simulink model "vehicle_svpwm"  (R2021a)
settings: Solver=VariableStepAuto  StartTime=0  StopTime=50  RelTol=1e-3
values from neighbouring files (symbols this model uses):
  Ld = 0.3e-3    (= 0.0003)    [PMSM_paramaters.m]
  Lq = 0.4e-3    (= 0.0004)    [PMSM_paramaters.m]
  P = 4    [PMSM_paramaters.m]
  Pm = 0.15    [PMSM_paramaters.m]
  Rs = 0.03    [PMSM_paramaters.m]
  T_lookup = [289,289,0]    [PMSM_paramaters.m]
  Torque = 289    [PMSM_paramaters.m]
  Ts = 1e-2    (= 0.01)    [PMSM_paramaters.m]
undefined symbols (not defined in the file or in its folder): sigbuilder_block
libraries: spsSeriesRLCBranchLib x18, spsMosfetLib x8, simulink x7, spsCurrentMeasurementLib x6, spsVoltageMeasurementLib x4, spsDCVoltageSourceLib x3, spsGroundLib x3, pid_lib x3, spsDiodeLib x2, spsRMSLib x2, autolibshared x1, spsTriangleGeneratorLib x1
(part 2 of 2)

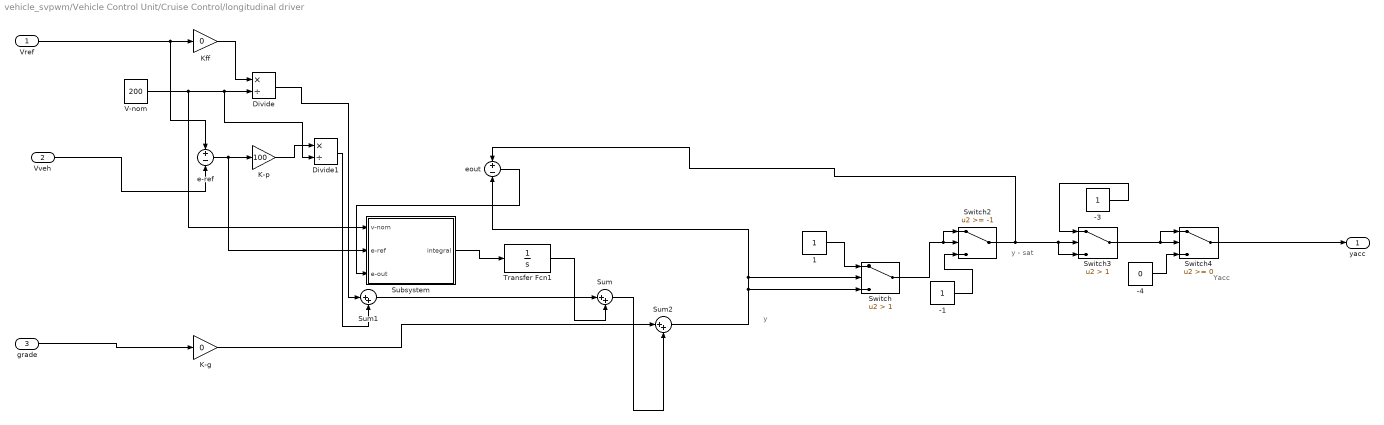
== system vehicle_svpwm/Vehicle Control Unit/Cruise Control/longitudinal driver ==
  note: Yacc
  note: y - sat
  note: y
  Vref : Inport
  Vveh : Inport  Port=2
  grade : Inport  Port=3
  -1 : Constant
  -3 : Constant
  -4 : Constant  Value=0
  1 : Constant
  Divide : Product  Inputs=*/
  Divide1 : Product  Inputs=*/
  K-g : Gain  Gain=0
  K-p : Gain  Gain=100
  Kff : Gain  Gain=0
  Subsystem : Subsystem
  Sum : Sum  Inputs=|++
  Sum1 : Sum  Inputs=|++
  Sum2 : Sum  Inputs=|++
  Switch : Switch  Criteria=u2 > Threshold  Threshold=1
  Switch2 : Switch  Threshold=-1
  Switch3 : Switch  Criteria=u2 > Threshold  Threshold=1
  Switch4 : Switch
  Transfer Fcn1 : TransferFcn  Denominator=[1 0]
  V-nom : Constant  Value=200
  e-ref : Sum  Inputs=+-
  eout : Sum  Inputs=+-
  yacc : Outport
  wires:
  1/1 -> Switch/1
  Switch4/1 -> yacc/1
  V-nom/1 -> Divide1/2, Divide/2, Subsystem/1(v-nom)
  Switch2/1 -> Switch3/3, Switch3/2, eout/1
  e-ref/1 -> Subsystem/2(e-ref), K-p/1
  Sum/1 -> Sum2/2
  -3/1 -> Switch3/1
  -4/1 -> Switch4/3
  Switch/1 -> Switch2/1, Switch2/2
  Divide/1 -> Sum1/1
  -1/1 -> Switch2/3
  Sum2/1 -> Switch/3, eout/2, Switch/2
  Vref/1 -> e-ref/1, Kff/1
  Subsystem/1(integral) -> Transfer Fcn1/1
  K-p/1 -> Divide1/1
  Sum1/1 -> Sum/1
  Switch3/1 -> Switch4/1, Switch4/2
  Transfer Fcn1/1 -> Sum/2
  Kff/1 -> Divide/1
  eout/1 -> Subsystem/3(e-out)
  Vveh/1 -> e-ref/2
  K-g/1 -> Sum2/1
  Divide1/1 -> Sum1/2
  grade/1 -> K-g/1

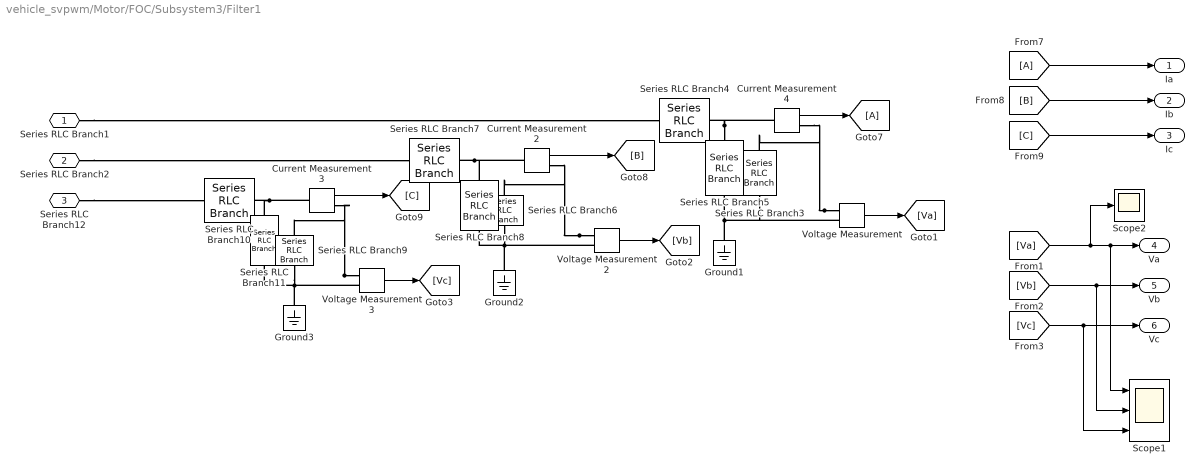
== system vehicle_svpwm/Motor/FOC/Subsystem3/Filter1 ==
  Current Measurement2 : spsCurrentMeasurementLib/Current Measurement  PhasorSimulation=off  OutputType=Complex  PSBequivalent=0
  Current Measurement3 : spsCurrentMeasurementLib/Current Measurement  PhasorSimulation=off  OutputType=Complex  PSBequivalent=0
  Current Measurement4 : spsCurrentMeasurementLib/Current Measurement  PhasorSimulation=off  OutputType=Complex  PSBequivalent=0
  Ground1 : spsGroundLib/Ground  LConnTagsString=a
  Ground2 : spsGroundLib/Ground  LConnTagsString=a
  Ground3 : spsGroundLib/Ground  LConnTagsString=a
  Scope1 : Scope  NumInputPorts=3
  Scope2 : Scope
  Series RLC Branch10 : spsSeriesRLCBranchLib/Series RLC Branch  LConnTagsString=__new0  RConnTagsString=__new0  BranchType=L  Resistance=1  Inductance=1e-3  SetiL0=off  InitialCurrent=0  Capacitance=1e-6  Setx0=off  InitialVoltage=0  Measurements=None
  Series RLC Branch11 : spsSeriesRLCBranchLib/Series RLC Branch  LConnTagsString=__new0  RConnTagsString=__new0  BranchType=C  Resistance=1  Inductance=1e-3  SetiL0=off  InitialCurrent=0  Capacitance=1000e-6  Setx0=off  InitialVoltage=0  Measurements=None
  Series RLC Branch3 : spsSeriesRLCBranchLib/Series RLC Branch  LConnTagsString=__new0  RConnTagsString=__new0  BranchType=R  Resistance=0.5  Inductance=1e-3  SetiL0=off  InitialCurrent=0  Capacitance=1e-6  Setx0=off  InitialVoltage=0  Measurements=None
  Series RLC Branch4 : spsSeriesRLCBranchLib/Series RLC Branch  LConnTagsString=__new0  RConnTagsString=__new0  BranchType=L  Resistance=1  Inductance=1e-3  SetiL0=off  InitialCurrent=0  Capacitance=1e-6  Setx0=off  InitialVoltage=0  Measurements=None
  Series RLC Branch5 : spsSeriesRLCBranchLib/Series RLC Branch  LConnTagsString=__new0  RConnTagsString=__new0  BranchType=C  Resistance=1  Inductance=1e-3  SetiL0=off  InitialCurrent=0  Capacitance=1000e-6  Setx0=off  InitialVoltage=0  Measurements=None
  Series RLC Branch6 : spsSeriesRLCBranchLib/Series RLC Branch  LConnTagsString=__new0  RConnTagsString=__new0  BranchType=R  Resistance=0.5  Inductance=1e-3  SetiL0=off  InitialCurrent=0  Capacitance=1e-6  Setx0=off  InitialVoltage=0  Measurements=None
  Series RLC Branch7 : spsSeriesRLCBranchLib/Series RLC Branch  LConnTagsString=__new0  RConnTagsString=__new0  BranchType=L  Resistance=1  Inductance=1e-3  SetiL0=off  InitialCurrent=0  Capacitance=1e-6  Setx0=off  InitialVoltage=0  Measurements=None
  Series RLC Branch8 : spsSeriesRLCBranchLib/Series RLC Branch  LConnTagsString=__new0  RConnTagsString=__new0  BranchType=C  Resistance=1  Inductance=1e-3  SetiL0=off  InitialCurrent=0  Capacitance=1000e-6  Setx0=off  InitialVoltage=0  Measurements=None
  Series RLC Branch9 : spsSeriesRLCBranchLib/Series RLC Branch  LConnTagsString=__new0  RConnTagsString=__new0  BranchType=R  Resistance=0.5  Inductance=1e-3  SetiL0=off  InitialCurrent=0  Capacitance=1e-6  Setx0=off  InitialVoltage=0  Measurements=None
  Voltage Measurement : spsVoltageMeasurementLib/Voltage Measurement  PhasorSimulation=off  OutputType=Complex  PSBequivalent=0
  Voltage Measurement2 : spsVoltageMeasurementLib/Voltage Measurement  PhasorSimulation=off  OutputType=Complex  PSBequivalent=0
  Voltage Measurement3 : spsVoltageMeasurementLib/Voltage Measurement  PhasorSimulation=off  OutputType=Complex  PSBequivalent=0
  Series RLC Branch1 : PMIOPort  Side=Left
  Series RLC Branch2 : PMIOPort  Port=2  Side=Left
  Series RLC Branch12 : PMIOPort  Port=3  Side=Left
  Ia : Outport
  Ib : Outport  Port=2
  Ic : Outport  Port=3
  Va : Outport  Port=4
  Vb : Outport  Port=5
  Vc : Outport  Port=6
  wires:
  [Vc] -> Vc/1, Scope1/3
  [Vb] -> Vb/1, Scope1/2
  [Va] -> Va/1, Scope1/1, Scope2/1
  [C] -> Ic/1
  Current Measurement4/1 -> [A]
  Voltage Measurement3/1 -> [Vc]
  [A] -> Ia/1
  Current Measurement3/1 -> [C]
  Voltage Measurement/1 -> [Va]
  [B] -> Ib/1
  Current Measurement2/1 -> [B]
  Voltage Measurement2/1 -> [Vb]
  connections:
  Series RLC Branch1/RConn1 -- Series RLC Branch4/LConn1
  Series RLC Branch2/RConn1 -- Series RLC Branch7/LConn1
  Voltage Measurement/LConn1 -- Series RLC Branch3/LConn1 -- Current Measurement4/RConn1
  Voltage Measurement2/LConn1 -- Series RLC Branch6/LConn1 -- Current Measurement2/RConn1
  Series RLC Branch12/RConn1 -- Series RLC Branch10/LConn1
  Voltage Measurement3/LConn1 -- Series RLC Branch9/LConn1 -- Current Measurement3/RConn1
  Series RLC Branch7/RConn1 -- Current Measurement2/LConn1 -- Series RLC Branch8/LConn1
  Ground1/LConn1 -- Series RLC Branch3/RConn1 -- Voltage Measurement/LConn2 -- Series RLC Branch5/RConn1
  Series RLC Branch9/RConn1 -- Voltage Measurement3/LConn2 -- Ground3/LConn1 -- Series RLC Branch11/RConn1
  Series RLC Branch5/LConn1 -- Current Measurement4/LConn1 -- Series RLC Branch4/RConn1
  Series RLC Branch6/RConn1 -- Ground2/LConn1 -- Voltage Measurement2/LConn2 -- Series RLC Branch8/RConn1
  Series RLC Branch10/RConn1 -- Series RLC Branch11/LConn1 -- Current Measurement3/LConn1

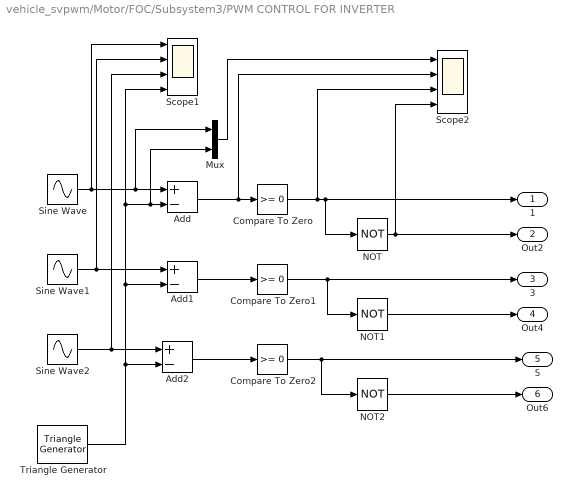
== system vehicle_svpwm/Motor/FOC/Subsystem3/PWM CONTROL FOR INVERTER ==
  Add : Sum  Inputs=+-
  Add1 : Sum  Inputs=+-
  Add2 : Sum  Inputs=+-
  Compare To Zero : simulink/Logic and Bit Operations/Compare To Zero  relop=>=  OutDataTypeStr=boolean
  Compare To Zero1 : simulink/Logic and Bit Operations/Compare To Zero  relop=>=  OutDataTypeStr=boolean
  Compare To Zero2 : simulink/Logic and Bit Operations/Compare To Zero  relop=>=  OutDataTypeStr=boolean
  Mux : Mux  Inputs=2
  NOT : Logic  Operator=NOT  IconShape=distinctive  AllPortsSameDT=off  OutDataTypeStr=boolean
  NOT1 : Logic  Operator=NOT  IconShape=distinctive  AllPortsSameDT=off  OutDataTypeStr=boolean
  NOT2 : Logic  Operator=NOT  IconShape=distinctive  AllPortsSameDT=off  OutDataTypeStr=boolean
  Scope1 : Scope  NumInputPorts=4
  Scope2 : Scope  NumInputPorts=4
  Sine Wave : Sin  Frequency=2*pi*50  SampleTime=0
  Sine Wave1 : Sin  Frequency=2*pi*50  Phase=2*pi/3  SampleTime=0
  Sine Wave2 : Sin  Frequency=2*pi*50  Phase=-2*pi/3  SampleTime=0
  Triangle Generator : spsTriangleGeneratorLib/Triangle Generator  Freq=1e3  Phase=90  Ts=0
  1 : Outport
  Out2 : Outport  Port=2
  3 : Outport  Port=3
  Out4 : Outport  Port=4
  5 : Outport  Port=5
  Out6 : Outport  Port=6
  wires:
  Triangle Generator/1 -> Add2/2, Add1/2, Scope1/4, Mux/2, Add/2
  Add/1 -> Scope2/2, Compare To Zero/1
  Compare To Zero/1 -> Scope2/3, 1/1, NOT/1
  Sine Wave/1 -> Scope1/1, Mux/1, Add/1
  Sine Wave1/1 -> Scope1/2, Add1/1
  Compare To Zero1/1 -> 3/1, NOT1/1
  Add1/1 -> Compare To Zero1/1
  Add2/1 -> Compare To Zero2/1
  NOT/1 -> Out2/1, Scope2/4
  NOT2/1 -> Out6/1
  Sine Wave2/1 -> Scope1/3, Add2/1
  Mux/1 -> Scope2/1
  Compare To Zero2/1 -> 5/1, NOT2/1
  NOT1/1 -> Out4/1

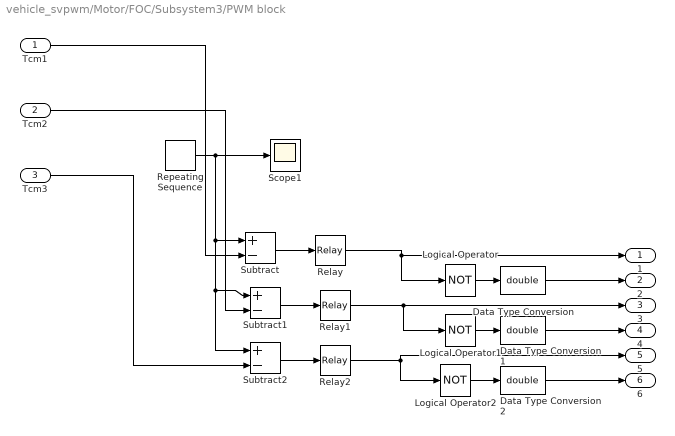
== system vehicle_svpwm/Motor/FOC/Subsystem3/PWM block ==
  Tcm1 : Inport
  Tcm2 : Inport  Port=2
  Tcm3 : Inport  Port=3
  Data Type Conversion : DataTypeConversion  OutDataTypeStr=double
  Data Type Conversion1 : DataTypeConversion  OutDataTypeStr=double
  Data Type Conversion2 : DataTypeConversion  OutDataTypeStr=double
  Logical Operator : Logic  Operator=NOT  AllPortsSameDT=off
  Logical Operator1 : Logic  Operator=NOT  AllPortsSameDT=off
  Logical Operator2 : Logic  Operator=NOT  AllPortsSameDT=off
  Relay : Relay
  Relay1 : Relay
  Relay2 : Relay
  Repeating Sequence : simulink/Sources/Repeating Sequence  rep_seq_t=[0 0.0001 0.0002]  rep_seq_y=[0 0.0001 0]
  Scope1 : Scope
  Subtract : Sum  Inputs=+-
  Subtract1 : Sum  Inputs=+-
  Subtract2 : Sum  Inputs=+-
  1 : Outport
  2 : Outport  Port=2
  3 : Outport  Port=3
  4 : Outport  Port=4
  5 : Outport  Port=5
  6 : Outport  Port=6
  wires:
  Subtract2/1 -> Relay2/1
  Relay2/1 -> 5/1, Logical Operator2/1
  Subtract1/1 -> Relay1/1
  Logical Operator1/1 -> Data Type Conversion1/1
  Tcm1/1 -> Subtract/2
  Relay/1 -> 1/1, Logical Operator/1
  Logical Operator/1 -> Data Type Conversion/1
  Repeating Sequence/1 -> Subtract/1, Subtract2/1, Subtract1/1, Scope1/1
  Logical Operator2/1 -> Data Type Conversion2/1
  Relay1/1 -> 3/1, Logical Operator1/1
  Data Type Conversion/1 -> 2/1
  Tcm2/1 -> Subtract1/2
  Subtract/1 -> Relay/1
  Data Type Conversion2/1 -> 6/1
  Tcm3/1 -> Subtract2/2
  Data Type Conversion1/1 -> 4/1

== system vehicle_svpwm/Motor/FOC/Subsystem3/Subsystem2 ==
  Ualfa : Inport
  Ubeta : Inport  Port=2
  Constant : Constant  Value=320
  Constant1 : Constant  Value=0.0002
  N1 : Subsystem
  Scope : Scope
  Scope1 : Scope
  Scope3 : Scope  NumInputPorts=2
  Scope6 : Scope
  Subsystem : Subsystem
  Subsystem1 : Subsystem
  X.Y.Z : Subsystem
  Tcm1 : Outport
  Tcm2 : Outport  Port=2
  Tcm3 : Outport  Port=3
  wires:
  Constant1/1 -> X.Y.Z/1(T), Subsystem1/3(T), Subsystem/5(T)
  Constant/1 -> X.Y.Z/4(Udc)
  N1/1(N) -> Subsystem1/4(N), Scope1/1, Subsystem/1(N)
  X.Y.Z/1(X) -> Subsystem/2(X)
  X.Y.Z/2(Y) -> Subsystem/3(Y)
  X.Y.Z/3(Z) -> Subsystem/4(Z)
  Subsystem1/1(Tcm1) -> Tcm1/1, Scope/1
  Subsystem1/2(Tcm2) -> Tcm2/1
  Subsystem1/3(Tcm3) -> Tcm3/1
  Ualfa/1 -> Scope3/1, X.Y.Z/2(Ualfa), N1/1(Ualfa)
  Subsystem/1(T1) -> Subsystem1/1(T1), Scope6/1
  Subsystem/2(T2) -> Subsystem1/2(T2)
  Ubeta/1 -> N1/2(Ubeta), X.Y.Z/3(Ubeta), Scope3/2

== system vehicle_svpwm/Motor/FOC/Subsystem3/Subsystem4 ==
  I : Inport
  V : Inport  Port=2
  IP : Inport  Port=3
  Display{,1..3} (4 alike) : Display
  Divide : Product  Inputs=*/
  Gain1 : Gain  Gain=100
  Product : Product
  RMS2 : spsRMSLib/RMS  TrueRMS=on  Freq=200  RMSInit=0  Ts=0
  RMS3 : spsRMSLib/RMS  TrueRMS=on  Freq=200  RMSInit=0  Ts=0
  Scope : Scope
  Scope1 : Scope
  Out1 : Outport
  Out2 : Outport  Port=2
  Out3 : Outport  Port=3
  Out5 : Outport  Port=4
  Out4 : Outport  Port=5
  wires:
  RMS3/1 -> Display1/1, Scope1/1, Out1/1, Product/2
  Gain1/1 -> Out4/1
  V/1 -> RMS2/1
  Product/1 -> Display3/1, Out3/1, Divide/1
  IP/1 -> Display2/1, Out5/1, Divide/2
  Divide/1 -> Gain1/1
  I/1 -> RMS3/1
  RMS2/1 -> Display/1, Scope/1, Out2/1, Product/1

== system vehicle_svpwm/Motor/FOC/Subsystem3/THREE PHASE INVERTER ==
  1 : Inport
  2 : Inport  Port=2
  3 : Inport  Port=3
  4 : Inport  Port=4
  5 : Inport  Port=5
  6 : Inport  Port=6
  Current Measurement : spsCurrentMeasurementLib/Current Measurement  PhasorSimulation=off  OutputType=Complex  PSBequivalent=0
  DC Voltage Source1 : spsDCVoltageSourceLib/DC Voltage Source  Amplitude=320  Measurements=None
  IGBT/Diode1 : spsIGBTDiodeLib/IGBT//Diode  Ron=1e-3  Rs=1e5  Cs=inf  Measurements=off
  Mosfet{,1..5} (6 alike) : spsMosfetLib/Mosfet  Ron=0.1  Lon=0  Rd=0.01  Vfd=0  IC=0  Rs=1e5  Cs=inf  Measurements=off
  Subsystem1 : Subsystem
  Voltage Measurement1 : spsVoltageMeasurementLib/Voltage Measurement  PhasorSimulation=off  OutputType=Complex  PSBequivalent=0
  A : PMIOPort  Side=Right
  B : PMIOPort  Port=2  Side=Right
  C : PMIOPort  Port=3  Side=Right
  Out1 : Outport
  wires:
  6/1 -> Mosfet5/1
  3/1 -> Mosfet1/1
  4/1 -> Mosfet4/1
  2/1 -> Mosfet3/1
  1/1 -> Mosfet/1
  5/1 -> Mosfet2/1
  Subsystem1/1(Out1) -> Out1/1
  Voltage Measurement1/1 -> Subsystem1/2(In2)
  Current Measurement/1 -> Subsystem1/1(In1)
  connections:
  Mosfet1/LConn1 -- Mosfet2/LConn1 -- Mosfet/LConn1 -- Current Measurement/RConn1
  B/RConn1 -- Mosfet4/LConn1 -- Mosfet1/RConn1
  A/RConn1 -- Mosfet3/LConn1 -- Mosfet/RConn1
  C/RConn1 -- Mosfet5/LConn1 -- Mosfet2/RConn1
  Mosfet3/RConn1 -- Mosfet5/RConn1 -- Mosfet4/RConn1 -- DC Voltage Source1/LConn1 -- Voltage Measurement1/LConn2
  Voltage Measurement1/LConn1 -- Current Measurement/LConn1 -- DC Voltage Source1/RConn1

== system vehicle_svpwm/Vehicle Control Unit/Cruise Control/longitudinal driver/Subsystem ==
  v-nom : Inport
  e-ref : Inport  Port=2
  e-out : Inport  Port=3
  Divide2 : Product  Inputs=*/
  K-aw : Gain  Gain=0
  Ki : Gain
  Sum2 : Sum  Inputs=|++
  integral : Outport
  wires:
  Divide2/1 -> Sum2/1
  v-nom/1 -> Divide2/2
  e-ref/1 -> Ki/1
  K-aw/1 -> Sum2/2
  Ki/1 -> Divide2/1
  e-out/1 -> K-aw/1
  Sum2/1 -> integral/1

== system vehicle_svpwm/Motor/FOC/Subsystem3/Subsystem2/N1 ==
  Ualfa : Inport
  Ubeta : Inport  Port=2
  Constant : Constant
  Constant1 : Constant  Value=0
  Gain : Gain  Gain=1.732
  Gain1 : Gain  Gain=-1.732
  Gain2 : Gain  Gain=2
  Gain3 : Gain  Gain=4
  Sum : Sum  Inputs=|-+
  Sum1 : Sum  Inputs=|-+
  Sum2 : Sum  Inputs=|+++
  Switch : Switch
  Switch1 : Switch
  Switch2 : Switch
  N : Outport
  wires:
  Ubeta/1 -> Switch/2, Sum/1, Sum1/1
  Constant/1 -> Switch/1, Switch2/1, Switch1/1
  Ualfa/1 -> Gain1/1, Gain/1
  Gain/1 -> Sum/2
  Sum/1 -> Switch1/2
  Sum1/1 -> Switch2/2
  Gain1/1 -> Sum1/2
  Constant1/1 -> Switch/3, Switch1/3, Switch2/3
  Switch1/1 -> Gain2/1
  Switch2/1 -> Gain3/1
  Gain2/1 -> Sum2/2
  Switch/1 -> Sum2/1
  Gain3/1 -> Sum2/3
  Sum2/1 -> N/1

== system vehicle_svpwm/Motor/FOC/Subsystem3/Subsystem2/Subsystem ==
  note: z
  note: y
  note: -z
  note: -x
  note: x
  note: -y
  note: y
  note: -x
  note: x
  note: z
  note: -y
  note: -z
  note: T1
  note: T2
  note: T
  note: T1
  note: T2
  N : Inport
  X : Inport  Port=2
  Y : Inport  Port=3
  Z : Inport  Port=4
  T : Inport  Port=5
  " " : Gain  Gain=-1
  "  " : Gain  Gain=-1
  "    " : Gain  Gain=-1
  Add : Sum
  Fcn : Fcn  Expr=u(3)-u(2)-u(1)
  Fcn1 : Fcn  Expr=u(1)*u(3)/(u(1)+u(2))
  Fcn2 : Fcn  Expr=u(2)*u(3)/(u(1)+u(2))
  Multiport Switch : MultiPortSwitch  Inputs=6
  Multiport Switch1 : MultiPortSwitch  Inputs=6
  Mux : Mux  Inputs=3
  Scope4 : Scope  NumInputPorts=3
  Switch : Switch
  Switch1 : Switch  Criteria=u2 > Threshold
  T1 : Outport
  T2 : Outport  Port=2
  wires:
  N/1 -> Multiport Switch1/1, Multiport Switch/1
  X/1 -> Multiport Switch1/4, Multiport Switch/6, " "/1
  Y/1 -> Multiport Switch1/2, Multiport Switch/3, "  "/1
  Z/1 -> Multiport Switch1/5, Multiport Switch/2, "    "/1
  "    "/1 -> Multiport Switch1/7, Multiport Switch/4
  "  "/1 -> Multiport Switch/7, Multiport Switch1/6
  " "/1 -> Multiport Switch/5, Multiport Switch1/3
  Multiport Switch/1 -> Mux/1, Switch/1, Add/2
  Multiport Switch1/1 -> Switch1/1, Mux/2, Add/1
  T/1 -> Mux/3
  Mux/1 -> Fcn/1, Fcn1/1, Fcn2/1
  Fcn/1 -> Switch/2, Switch1/2
  Fcn1/1 -> Switch/3
  Fcn2/1 -> Switch1/3
  Switch/1 -> T1/1, Scope4/1
  Switch1/1 -> T2/1, Scope4/2
  Add/1 -> Scope4/3

== system vehicle_svpwm/Motor/FOC/Subsystem3/Subsystem2/Subsystem1 ==
  note: Ta
  note: Tb
  note: Tc
  note: b
  note: a
  note: a
  note: c
  note: c
  note: b
  note: a
  note: c
  note: b
  note: b
  note: a
  note: c
  note: c
  note: b
  note: c
  note: a
  note: b
  note: a
  T1 : Inport
  T2 : Inport  Port=2
  T : Inport  Port=3
  N : Inport  Port=4
  Gain1 : Gain  Gain=1/4
  Gain2 : Gain  Gain=0.5
  Gain3 : Gain  Gain=0.5
  Multiport Switch : MultiPortSwitch  Inputs=6
  Multiport Switch1 : MultiPortSwitch  Inputs=6
  Multiport Switch2 : MultiPortSwitch  Inputs=6
  Subtract1 : Sum  Inputs=--+
  Subtract2 : Sum
  Subtract3 : Sum
  Tcm1 : Outport
  Tcm2 : Outport  Port=2
  Tcm3 : Outport  Port=3
  wires:
  T2/1 -> Gain2/1, Subtract1/2
  T/1 -> Subtract1/3
  T1/1 -> Gain3/1, Subtract1/1
  Gain3/1 -> Subtract2/1
  Subtract1/1 -> Gain1/1
  Gain1/1 -> Subtract2/2, Multiport Switch/3, Multiport Switch/4, Multiport Switch1/2, Multiport Switch1/6, Multiport Switch2/5, Multiport Switch2/7
  Subtract2/1 -> Subtract3/2, Multiport Switch/2, Multiport Switch/7, Multiport Switch1/4, Multiport Switch1/5, Multiport Switch2/3, Multiport Switch2/6
  Gain2/1 -> Subtract3/1
  N/1 -> Multiport Switch/1, Multiport Switch2/1, Multiport Switch1/1
  Multiport Switch/1 -> Tcm1/1
  Multiport Switch1/1 -> Tcm2/1
  Multiport Switch2/1 -> Tcm3/1
  Subtract3/1 -> Multiport Switch/5, Multiport Switch/6, Multiport Switch1/3, Multiport Switch1/7, Multiport Switch2/2, Multiport Switch2/4

== system vehicle_svpwm/Motor/FOC/Subsystem3/Subsystem2/X.Y.Z ==
  T : Inport
  Ualfa : Inport  Port=2
  Ubeta : Inport  Port=3
  Udc : Inport  Port=4
  Divide : Product  Inputs=**/
  Divide1 : Product  Inputs=**/
  Divide2 : Product  Inputs=**/
  Gain : Gain  Gain=0.577
  Gain1 : Gain  Gain=1.732
  Gain2 : Gain  Gain=1.5
  Gain3 : Gain  Gain=1.5
  Subtract : Sum
  Subtract1 : Sum  Inputs=+-
  X : Outport
  Y : Outport  Port=2
  Z : Outport  Port=3
  wires:
  Gain/1 -> Subtract/1, Subtract1/1
  Gain1/1 -> Divide/1
  T/1 -> Divide2/2, Divide1/2, Divide/2
  Udc/1 -> Divide2/3, Divide1/3, Divide/3
  Ualfa/1 -> Subtract1/2, Subtract/2
  Subtract/1 -> Divide1/1
  Subtract1/1 -> Divide2/1
  Divide/1 -> X/1
  Divide1/1 -> Gain2/1
  Divide2/1 -> Gain3/1
  Gain2/1 -> Y/1
  Gain3/1 -> Z/1
  Ubeta/1 -> Gain1/1, Gain/1

== system vehicle_svpwm/Motor/FOC/Subsystem3/THREE PHASE INVERTER/Subsystem1 ==
  In1 : Inport
  In2 : Inport  Port=2
  Mean1 : spsMeanLib/Mean  Freq=50  Vinit=0  Ts=0
  Product1 : Product
  Scope5 : Scope
  Scope6 : Scope
  Out1 : Outport
  wires:
  Mean1/1 -> Product1/1
  In1/1 -> Mean1/1, Scope5/1
  Product1/1 -> Out1/1, Scope6/1
  In2/1 -> Product1/2
